simulink model "sgMdl_IO641_IO642_PROFIBUSLoopback"  (R2024b)
settings: Solver=FixedStepAuto  StartTime=0.0  StopTime=inf  RelTol=1e-3  EnableMultiTasking=on
undefined symbols (not defined in the file): C, Ts
libraries: slrealtimeutilitieslib x4, speedgoatlib_IO641 x3, speedgoatlib_IO642 x3, simulink x2, speedgoatlib_shared x1
Description:
  | IO641 & IO642 - PROFIBUS Loopback
settings Model: ModifiedByFormat=Speedgoat  Creator=Speedgoat  LastModifiedBy=Speedgoat
settings SolverCC: ConcurrentTasks=on  AlgebraicLoopSolver=TrustRegion  PositivePriorityOrder=on  AutoInsertRateTranBlk=on  InsertRTBMode=Never (minimum delay)
settings DataIOCC: SaveFormat=Array  SaveState=on  SignalLoggingName=logsOut
settings OptimizationCC: BlockReduction=off  BooleanDataType=off  OptimizeBlockIOStorage=off  BufferReuse=off  GlobalBufferReuse=off  ExpressionFolding=off  LocalBlockOutputs=off  InitFltsAndDblsToZero=on  OptimizeDataStoreBuffers=off  BusAssignmentInplaceUpdate=off
settings DebuggingCC: SaveWithParameterizedLinksMsg=none  UnderspecifiedInitializationDetection=Classic  MergeDetectMultiDrivingBlocksExec=none  CheckExecutionContextPreStartOutputMsg=on  SignalResolutionControl=TryResolveAllWithWarning  TasksWithSamePriorityMsg=none  UnconnectedInputMsg=warning  UnconnectedOutputMsg=warning  UnconnectedLineMsg=warning  SFUnexpectedBacktrackingDiag=warning  SFNoUnconditionalDefaultTransitionDiag=warning  SFExecutionAtInitializationDiag=none  ArithmeticOperatorsInVariantConditions=warning
settings HardwareCC: ProdBitPerLong=64  ProdLongLongMode=on  ProdHWDeviceType=Intel->x86-64 (Linux 64)
settings ModelReferenceCC: EnableRefExpFcnMdlSchedulingChecks=on  PropagateSignalLabelsOutOfModel=off
settings SFSimCC: SimUseLocalCustomCode=off  SimTargetLang=C++
settings RTWCC: Description=Speedgoat Real-Time Target Machine  SystemTargetFile=speedgoat.tlc  TemplateMakefile=slrealtime_default_tmf  RTWUseLocalCustomCode=off  Toolchain=Simulink Real-Time Toolchain  BuildConfiguration=Faster Runs  TargetLang=C++  GPUComputeCapability=3.5  DLArmComputeVersion=19.05
settings CodeAppCC: StateflowObjectComments=on
settings SimulinkRealTimeTargetCC: SubcomponentCodeInterfacePackaging=Reusable function  MATLABClassNameForMDSCustomization=Simulink.SoftwareTarget.GRTCustomization  InstructionSetFMA=off  LogToMDFFile=off  SLRTFileLogMaxRuns=10  UseGCCFastMath=on
settings ConfigComp: CovMetricSettings=dw  CovSaveCumulativeToWorkspaceVar=on  CovSaveSingleToWorkspaceVar=on  CovExternalEMLEnable=off  CovSFcnEnable=off  CovBoundaryAbsTol=1.0e-5

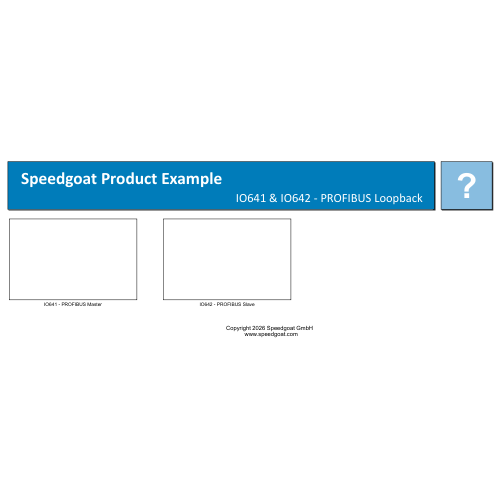
[thumbnail: Simulink's stored preview of the top-level diagram]
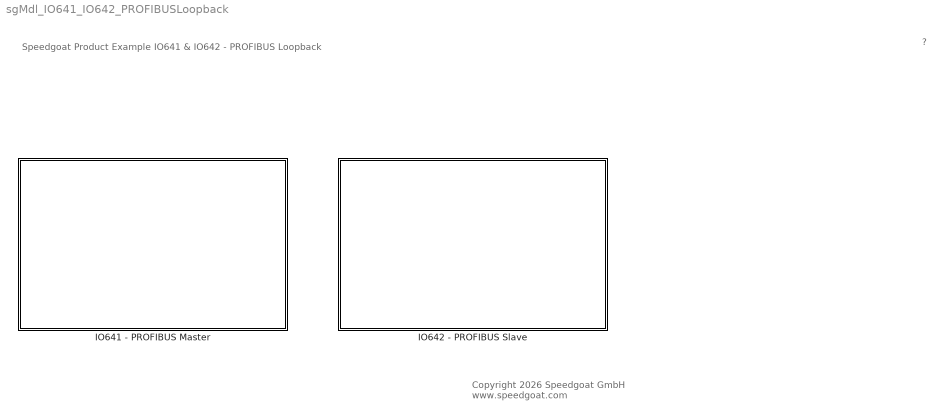
== system sgMdl_IO641_IO642_PROFIBUSLoopback ==
  note: Speedgoat Product Example
      | IO641 & IO642 - PROFIBUS Loopback
  note: ?
  note: Copyright 2026 Speedgoat GmbH
      |  www.speedgoat.com
  IO641 - PROFIBUS Master : Subsystem
  IO642 - PROFIBUS Slave : Subsystem

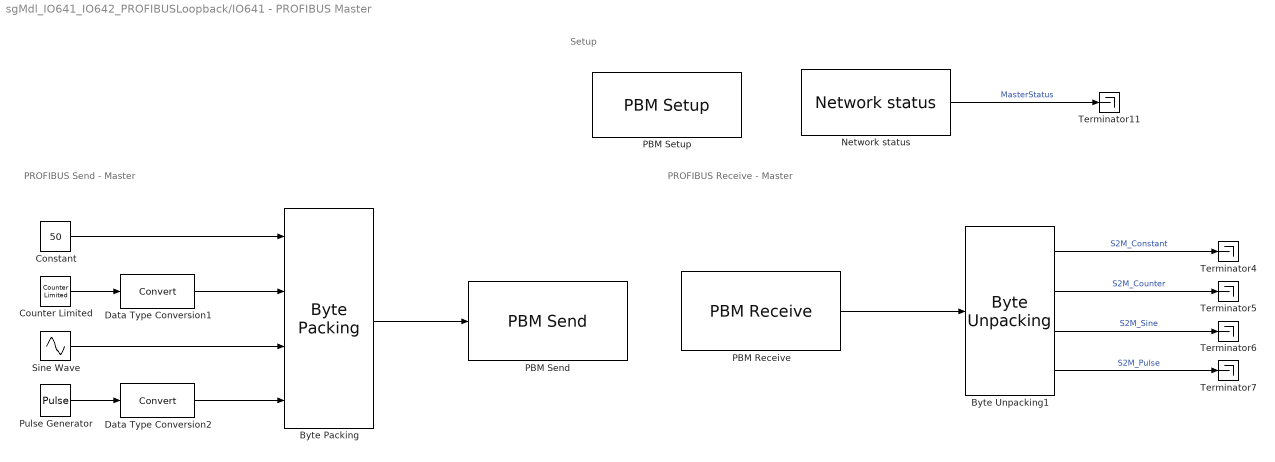
== system sgMdl_IO641_IO642_PROFIBUSLoopback/IO641 - PROFIBUS Master ==
  note: PROFIBUS Receive - Master
  note: PROFIBUS Send - Master
  note: Setup
  Byte Packing : slrealtimeutilitieslib/Byte Packing  MaskPackedDataType=uint8  MaskUnpackedDataTypes={'int8','uint16','double','int32'}  MaskAlignment=1
  Byte Unpacking1 : slrealtimeutilitieslib/Byte Unpacking  MaskUnpackedDataTypes={'int16','uint32','single','uint8'}  MaskUnpackedDataSizes={[1],[1],[1],[1]}  MaskAlignment=1
  Constant : Constant  Value=50  OutDataTypeStr=Inherit: Inherit via back propagation  SampleTime=Ts
  Counter Limited : simulink/Sources/Counter Limited  uplimit=100  tsamp=Ts/Ts/10
  Data Type Conversion1 : DataTypeConversion  SaturateOnIntegerOverflow=off  RndMeth=Floor
  Data Type Conversion2 : DataTypeConversion  SaturateOnIntegerOverflow=off  RndMeth=Floor
  Network status : speedgoatlib_shared/IO64X/Network status  id=1  get_status=on  set_status=off  timeout=0.01  ts=Ts
  PBM Receive : speedgoatlib_IO641/PBM Receive  id=1  portType=1 port with n element vector of type UINT8  inputOutput=11  sampleTime=Ts
      settings: SourceProductName=IO641 PROFIBUS DP Master
  PBM Send : speedgoatlib_IO641/PBM Send  id=1  portType=1 port with n element vector of type UINT8  inputOutput=15  sampleTime=Ts
      settings: SourceProductName=IO641 PROFIBUS DP Master
  PBM Setup : speedgoatlib_IO641/PBM Setup  id=1  driveLetter=C:  configurationMode=Configuration file  mode=Polling mode  sampleTime=-1  pciSlot=-1  quantityOfAcyclicObjects=0  qtyMods=[1,0,0]  ConfigFile=which('IO641_IO642_Loopback_m.nxd')  protocol=IO641  firmware=PROFIBUS DP Master
      settings: SourceProductName=IO641 PROFIBUS DP Master
  Pulse Generator : DiscretePulseGenerator  Amplitude=100  Period=2*1/Ts  PulseWidth=1/Ts  SampleTime=Ts
  Sine Wave : Sin  Amplitude=100  Frequency=2*pi  Phase=pi  SampleTime=Ts
  Terminator{4..7,11} (5 alike) : Terminator
  wires:
  Sine Wave/1 -> Byte Packing/3
  Counter Limited/1 -> Data Type Conversion1/1
  Constant/1 -> Byte Packing/1
  Byte Unpacking1/1 -> Terminator4/1  "S2M_Constant"
  Byte Unpacking1/2 -> Terminator5/1  "S2M_Counter"
  Byte Unpacking1/3 -> Terminator6/1  "S2M_Sine"
  Byte Unpacking1/4 -> Terminator7/1  "S2M_Pulse"
  Data Type Conversion1/1 -> Byte Packing/2
  Data Type Conversion2/1 -> Byte Packing/4
  Byte Packing/1 -> PBM Send/1
  PBM Receive/1 -> Byte Unpacking1/1
  Pulse Generator/1 -> Data Type Conversion2/1
  Network status/1 -> Terminator11/1  "MasterStatus"

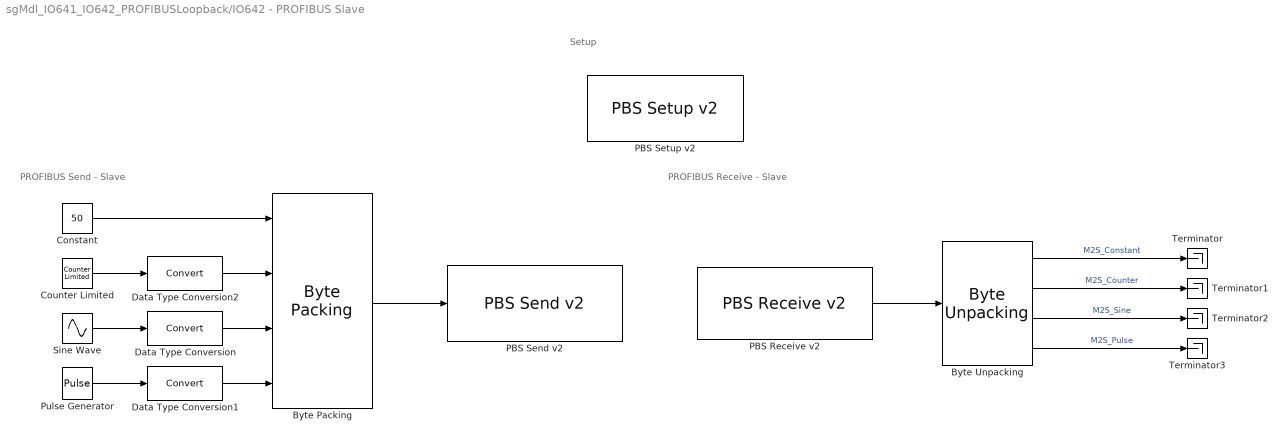
== system sgMdl_IO641_IO642_PROFIBUSLoopback/IO642 - PROFIBUS Slave ==
  note: PROFIBUS Receive - Slave
  note: PROFIBUS Send - Slave
  note: Setup
  Byte Packing : slrealtimeutilitieslib/Byte Packing  MaskPackedDataType=uint8  MaskUnpackedDataTypes={'int16','uint32','single','uint8'}  MaskAlignment=1
  Byte Unpacking : slrealtimeutilitieslib/Byte Unpacking  MaskUnpackedDataTypes={'int8','uint16','double','int32'}  MaskUnpackedDataSizes={[1],[1],[1],[1]}  MaskAlignment=1
  Constant : Constant  Value=50  OutDataTypeStr=Inherit: Inherit via back propagation  SampleTime=Ts
  Counter Limited : simulink/Sources/Counter Limited  uplimit=100  tsamp=Ts/Ts/10
  Data Type Conversion : DataTypeConversion  SaturateOnIntegerOverflow=off  RndMeth=Floor
  Data Type Conversion1 : DataTypeConversion  SaturateOnIntegerOverflow=off  RndMeth=Floor
  Data Type Conversion2 : DataTypeConversion  SaturateOnIntegerOverflow=off  RndMeth=Floor
  "PBS Receive v2 " : speedgoatlib_IO642/PBS Receive v2   id=2  len=15  ts=Ts
      settings: SourceProductName="IO642  PROFIBUS DP Slave"
  "PBS Send v2 " : speedgoatlib_IO642/PBS Send v2   id=2  len=11  ts=-1
      settings: SourceProductName="IO642  PROFIBUS DP Slave"
  "PBS Setup v2 " : speedgoatlib_IO642/PBS Setup v2   id=2  drive=C:  slot=-1  busStartup=Automatic  busAddress=2  manualConfig=off  identNumber=hex2dec('0B69')  baudRate=Auto detect  watchdogTime=0  ioStatus=None  ioConfiguration=on  ioData=0  ioDataSwap=off  dpv1Enable=on  syncSupported=on  freezeSupported=on  failSafeSupported=off  alarmSap50=on  addressChange=off  alarmModeNoSeq=off  protocol=IO642  firmware=PROFIBUS DP Slave
      settings: SourceProductName="IO642  PROFIBUS DP Slave"
  Pulse Generator : DiscretePulseGenerator  Amplitude=100  Period=2*1/Ts  PulseWidth=1/Ts  SampleTime=Ts
  Sine Wave : Sin  Amplitude=100  Frequency=2*pi  Phase=pi  SampleTime=Ts
  Terminator{,1..3} (4 alike) : Terminator
  wires:
  "PBS Receive v2 "/1 -> Byte Unpacking/1
  Byte Packing/1 -> "PBS Send v2 "/1
  Byte Unpacking/1 -> Terminator/1  "M2S_Constant"
  Byte Unpacking/2 -> Terminator1/1  "M2S_Counter"
  Byte Unpacking/3 -> Terminator2/1  "M2S_Sine"
  Byte Unpacking/4 -> Terminator3/1  "M2S_Pulse"
  Constant/1 -> Byte Packing/1
  Counter Limited/1 -> Data Type Conversion2/1
  Sine Wave/1 -> Data Type Conversion/1
  Data Type Conversion/1 -> Byte Packing/3
  Data Type Conversion1/1 -> Byte Packing/4
  Data Type Conversion2/1 -> Byte Packing/2
  Pulse Generator/1 -> Data Type Conversion1/1
